simulink model "Q1B_model"  (R2018a)
settings: Solver=VariableStepAuto  StartTime=0.0  StopTime=250  RelTol=1e-3
settings Model: Creator=lab User  LastModifiedBy=lab User

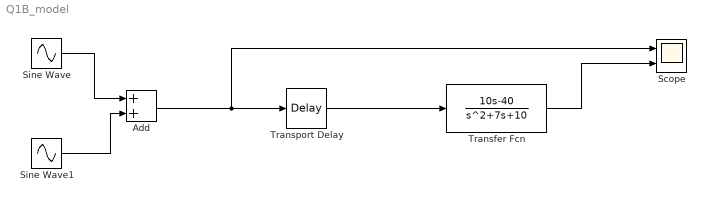
== system Q1B_model ==
  Add : Sum
  Scope : Scope  NumInputPorts=2
  Sine Wave : Sin  Amplitude=2  Frequency=4  SampleTime=0
  Sine Wave1 : Sin  Frequency=0.1  Phase=-1.5708  SampleTime=0
  Transfer Fcn : TransferFcn  Numerator=[10 -40]  Denominator=[1 7 10]
  Transport Delay : TransportDelay  DelayTime=3
  wires:
  Sine Wave/1 -> Add/1
  Sine Wave1/1 -> Add/2
  Add/1 -> Scope/1, Transport Delay/1
  Transport Delay/1 -> Transfer Fcn/1
  Transfer Fcn/1 -> Scope/2
